simulink model "task2_3"  (R2015b)
settings: Solver=ode45  StartTime=tstart  StopTime=tstop  RelTol=1e-3
values from neighbouring files (symbols this model uses):
  c = 0    [matlab.mat]    (also in run.m; run_2_3.m = 1; test.m)
  delta_max = 0.436332312999    [matlab.mat]
  DELTA_s = 0.01    [matlab.mat]    (also in run_2_3.m = 1)
  k_b0 = 0.009    [matlab.mat]
  kd_psi = 500    [matlab.mat]
  ki_psi = 0.8    [matlab.mat]
  Ki_u = 0.0005    [matlab.mat]
  kp_psi = 190    [matlab.mat]
  Kp_u = 10    [matlab.mat]
  n_c_k = 1.02    [matlab.mat]
  n_c_max = 8.9    [matlab.mat]
  n_dot_max = 0.0436332312999    [matlab.mat]
  psi0 = 0    [matlab.mat]    (also in run.m; run_2_3.m; test.m)
  r0 = 0    [matlab.mat]    (also in run.m; run_2_3.m; test.m)
  tsamp = 10    [matlab.mat]    (also in run.m; run_2_3.m; test.m)
  Ua_MAX = 1    [matlab.mat]
  v0 = [6.63 0]    [matlab.mat]    (also in run.m = [6.63 0]'; run_2_3.m = [6.63 0]'; test.m = [6.63 0]')
  WP = [-600  4680  7662  10644  13626; 0  3880  2248  3878  2246]    [matlab.mat]
undefined symbols (not defined in the file or in its folder): Kd_u, msfartoystyring, N_u
undefined symbols (not defined in the file): p0
libraries: simulink x1
settings Model: ExtModeAutoUpdateStatusClock=off  Creator=christh  LastModifiedBy=ShivJeet
settings DataIOCC: SaveFormat=Array  SignalLoggingSaveFormat=ModelDataLogs
settings OptimizationCC: ExpressionDepthLimit=2147483647  InitFltsAndDblsToZero=on
settings DebuggingCC: UnderspecifiedInitializationDetection=Classic  MergeDetectMultiDrivingBlocksExec=none  SolverPrmCheckMsg=warning  FcnCallInpInsideContextMsg=UseLocalSettings  StateNameClashWarn=warning
settings HardwareCC: ProdBitPerPointer=32  ProdLargestAtomicFloat=None  ProdIntDivRoundTo=Undefined  ProdEndianess=Unspecified  ProdWordSize=32  ProdHWDeviceType=32-bit Generic
settings GRTTargetCC: GeneratePreprocessorConditionals=Disable all  CombineOutputUpdateFcns=off  GRTInterface=on
settings ConfigComp: CovModelRefEnable=Off

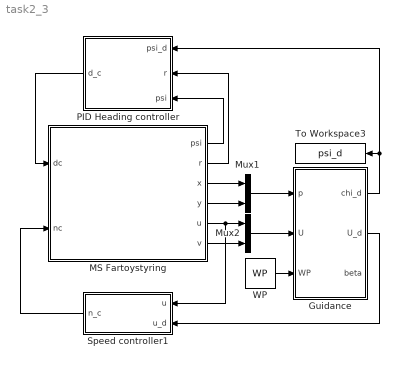
== system task2_3 ==
  Guidance : Subsystem
  MS Fartoystyring : Subsystem  mask(MS Fartoystyring for Assignment 3 G&C){x0=p0(1), y0=p0(2), u0=v0(1), v0=v0(2), psi0=psi0, r0=r0, c=c}
      mask prompts: x0 "x(t0) (m)"; y0 "y(t0) (m)"; u0 "u(t0) (m/s)"; v0 "v(t0) (m/s)"; psi0 "psi(t0) (rad)"; r0 "r(t0) (rad/s)"; c "current (0 or 1)"
      mask help:
      | Block corresponding to Figure 1 in the assignment text. Gives the response of the ship.
      |
      | The design speed of MS Fartoystyring is u=8.23 m/s.
      |
      | Input:
      | dc: commanded rudder (rad), dmax=25*pi/180
      | nc: commanded shaft speed (rad/s), nmax=85*2*pi/60
      |
      | Output:
      | x: north pos (m)
      | y: east pos (m)
      | u: surge (m/s)
      | v: sway (m/s)
      | psi: heading (rad)
      | r: yaw (rad/s)
      mask Help: Comments, bugs and help requests can be directed to the TA. Email on course website.
  Mux1 : Mux  Inputs=2
  Mux2 : Mux  Inputs=2
  PID Heading controller : Subsystem
  Speed controller1 : Subsystem
  To Workspace3 : ToWorkspace  VariableName=psi_d  SampleTime=tsamp
  WP : Constant  Value=WP
  wires:
  MS Fartoystyring/1(psi) -> PID Heading controller/3(psi)
  MS Fartoystyring/2(r) -> PID Heading controller/2(r)
  Speed controller1/1(n_c) -> MS Fartoystyring/2(nc)
  MS Fartoystyring/3(x) -> Mux1/1
  MS Fartoystyring/4(y) -> Mux1/2
  Mux1/1 -> Guidance/1(p)
  MS Fartoystyring/5(u) -> Speed controller1/1(u), Mux2/1
  PID Heading controller/1(d_c) -> MS Fartoystyring/1(dc)
  MS Fartoystyring/6(v) -> Mux2/2
  Mux2/1 -> Guidance/2(U)
  WP/1 -> Guidance/3(WP)
  Guidance/2(U_d) -> Speed controller1/2(u_d)
  Guidance/1(chi_d) -> PID Heading controller/1(psi_d), To Workspace3/1

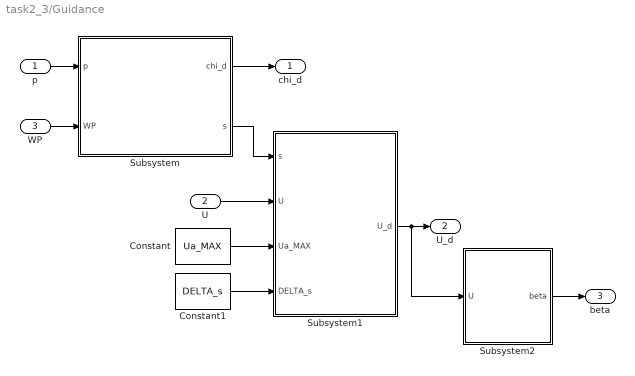
== system task2_3/Guidance ==
  p : Inport
  U : Inport  Port=2
  WP : Inport  Port=3
  Constant : Constant  Value=Ua_MAX
  Constant1 : Constant  Value=DELTA_s
  Subsystem : Subsystem
  Subsystem1 : Subsystem
  Subsystem2 : Subsystem
  chi_d : Outport
  U_d : Outport  Port=2
  beta : Outport  Port=3
  wires:
  U/1 -> Subsystem1/2("U ")
  Subsystem1/1(U_d) -> U_d/1, Subsystem2/1("U ")
  p/1 -> Subsystem/1(p)
  WP/1 -> Subsystem/2(WP)
  Subsystem/1(chi_d) -> chi_d/1
  Constant/1 -> Subsystem1/3(Ua_MAX)
  Subsystem/2(s) -> Subsystem1/1(s)
  Constant1/1 -> Subsystem1/4(DELTA_s)
  Subsystem2/1(beta) -> beta/1

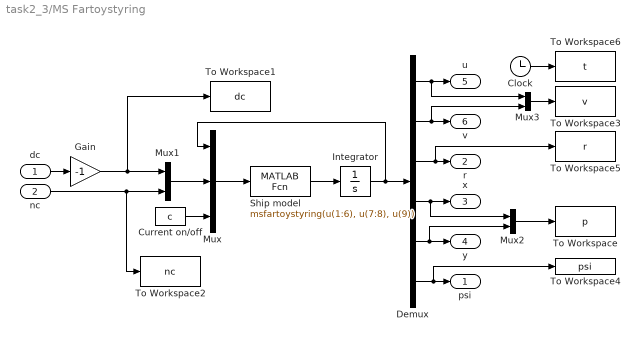
== system task2_3/MS Fartoystyring ==
  dc : Inport
  nc : Inport  Port=2
  Clock : Clock
  Current on/off : Constant  Value=c
  Demux : Demux  Outputs=6
  Gain : Gain  Gain=-1
  Integrator : Integrator  InitialCondition=[u0 v0 r0 x0 y0 psi0]'
  Mux : Mux  Inputs=3
  Mux1 : Mux  Inputs=2
  Mux2 : Mux  Inputs=2
  Mux3 : Mux  Inputs=2
  Ship model : MATLABFcn  MATLABFcn=msfartoystyring(u(1:6), u(7:8), u(9))  OutputDimensions=6
  To Workspace : ToWorkspace  VariableName=p  SampleTime=tsamp
  To Workspace1 : ToWorkspace  VariableName=dc  SampleTime=tsamp
  To Workspace2 : ToWorkspace  VariableName=nc  SampleTime=tsamp
  To Workspace3 : ToWorkspace  VariableName=v  SampleTime=tsamp
  To Workspace4 : ToWorkspace  VariableName=psi  SampleTime=tsamp
  To Workspace5 : ToWorkspace  VariableName=r  SampleTime=tsamp
  To Workspace6 : ToWorkspace  VariableName=t  SampleTime=tsamp
  psi : Outport
  r : Outport  Port=2
  x : Outport  Port=3
  y : Outport  Port=4
  u : Outport  Port=5
  v : Outport  Port=6
  wires:
  Integrator/1 -> Mux/1, Demux/1
  Mux1/1 -> Mux/2
  dc/1 -> Gain/1
  nc/1 -> Mux1/2, To Workspace2/1
  Demux/1 -> Mux3/1, u/1
  Demux/2 -> Mux3/2, v/1
  Demux/3 -> To Workspace5/1, r/1
  Demux/4 -> Mux2/1, x/1
  Demux/5 -> y/1, Mux2/2
  Demux/6 -> To Workspace4/1, psi/1
  Current on/off/1 -> Mux/3
  Ship model/1 -> Integrator/1
  Mux/1 -> Ship model/1
  Mux2/1 -> To Workspace/1
  Clock/1 -> To Workspace6/1
  Mux3/1 -> To Workspace3/1
  Gain/1 -> To Workspace1/1, Mux1/1

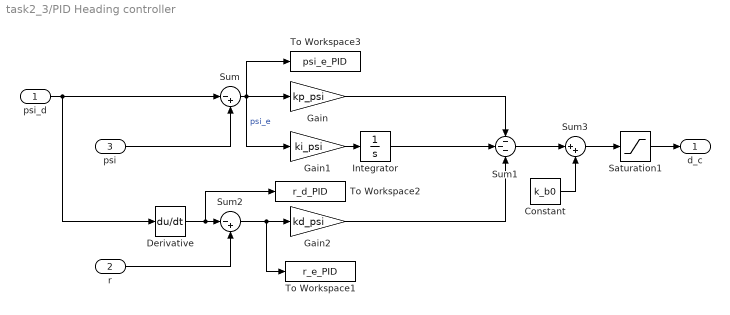
== system task2_3/PID Heading controller ==
  psi_d : Inport
  r : Inport  Port=2
  psi : Inport  Port=3
  Constant : Constant  Value=k_b0
  Derivative : Derivative
  Gain : Gain  Gain=kp_psi
  Gain1 : Gain  Gain=ki_psi
  Gain2 : Gain  Gain=kd_psi
  Integrator : Integrator
  Saturation1 : Saturate  UpperLimit=delta_max  LowerLimit=-delta_max
  Sum : Sum  Inputs=|-+
  Sum1 : Sum  Inputs=---
  Sum2 : Sum  Inputs=|-+
  Sum3 : Sum  Inputs=|++
  To Workspace1 : ToWorkspace  VariableName=r_e_PID  SampleTime=tsamp
  To Workspace2 : ToWorkspace  VariableName=r_d_PID  SampleTime=tsamp
  To Workspace3 : ToWorkspace  VariableName=psi_e_PID  SampleTime=tsamp
  d_c : Outport
  wires:
  psi_d/1 -> Derivative/1, Sum/1
  Saturation1/1 -> d_c/1
  Sum3/1 -> Saturation1/1
  psi/1 -> Sum/2
  Sum/1 -> Gain1/1, Gain/1, To Workspace3/1  "psi_e"
  Gain1/1 -> Integrator/1
  Gain/1 -> Sum1/1
  Integrator/1 -> Sum1/2
  Gain2/1 -> Sum1/3
  Sum1/1 -> Sum3/1
  Constant/1 -> Sum3/2
  Sum2/1 -> To Workspace1/1, Gain2/1
  r/1 -> Sum2/2
  Derivative/1 -> To Workspace2/1, Sum2/1

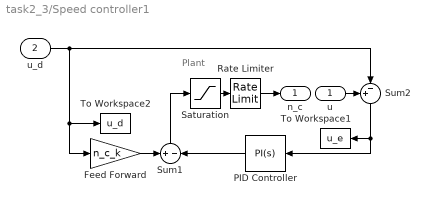
== system task2_3/Speed controller1 ==
  note: Plant
  u : Inport
  u_d : Inport  Port=2
  Feed Forward : Gain  Gain=n_c_k
  PID Controller : simulink/Continuous/PID Controller  Controller=PI  TimeDomain=Continuous-time  SampleTime=-1  IntegratorMethod=Forward Euler  FilterMethod=Forward Euler  Form=Parallel  UseFilter=on  ControllerParametersSource=internal  P=Kp_u  I=Ki_u  D=Kd_u  N=N_u  InitialConditionSource=internal  InitialConditionForIntegrator=0  InitialConditionForFilter=0  ExternalReset=none  LimitOutput=off  UpperSaturationLimit=inf  LowerSaturationLimit=-inf  LinearizeAsGain=on  AntiWindupMode=none  Kb=1  TrackingMode=off  Kt=1  PParamMin=[]  PParamMax=[]  IParamMin=[]  IParamMax=[]  DParamMin=[]  DParamMax=[]  NParamMin=[]  NParamMax=[]  KbParamMin=[]  KbParamMax=[]  KtParamMin=[]  KtParamMax=[]  POutMin=[]  POutMax=[]  IOutMin=[]  IOutMax=[]  DOutMin=[]  DOutMax=[]  NOutMin=[]  NOutMax=[]  KbOutMin=[]  KbOutMax=[]  KtOutMin=[]  KtOutMax=[]  IntegratorOutMin=[]  IntegratorOutMax=[]  FilterOutMin=[]  FilterOutMax=[]  SumOutMin=[]  SumOutMax=[]  SumI1OutMin=[]  SumI1OutMax=[]  SumI2OutMin=[]  SumI2OutMax=[]  SumI3OutMin=[]  SumI3OutMax=[]  SumDOutMin=[]  SumDOutMax=[]  SaturationOutMin=[]  SaturationOutMax=[]  IntegratorContinuousStateAttributes=''  IntegratorStateMustResolveToSignalObject=off  IntegratorRTWStateStorageClass=Auto  FilterContinuousStateAttributes=''  FilterStateMustResolveToSignalObject=off  FilterRTWStateStorageClass=Auto  DifferentiatorICPrevScaledInput=0  DifferentiatorOutMin=[]  DifferentiatorOutMax=[]
  Rate Limiter : RateLimiter  RisingSlewLimit=n_dot_max  FallingSlewLimit=-n_dot_max
  Saturation : Saturate  UpperLimit=n_c_max  LowerLimit=0.0001
  Sum1 : Sum  Inputs=+-
  Sum2 : Sum  Inputs=+-|
  To Workspace1 : ToWorkspace  VariableName=u_e  SampleTime=tsamp
  To Workspace2 : ToWorkspace  VariableName=u_d  SampleTime=tsamp
  n_c : Outport
  wires:
  Sum1/1 -> Saturation/1
  Saturation/1 -> Rate Limiter/1
  Rate Limiter/1 -> n_c/1
  u_d/1 -> Sum2/2, To Workspace2/1, Feed Forward/1
  Feed Forward/1 -> Sum1/1
  u/1 -> Sum2/1
  Sum2/1 -> PID Controller/1, To Workspace1/1
  PID Controller/1 -> Sum1/2

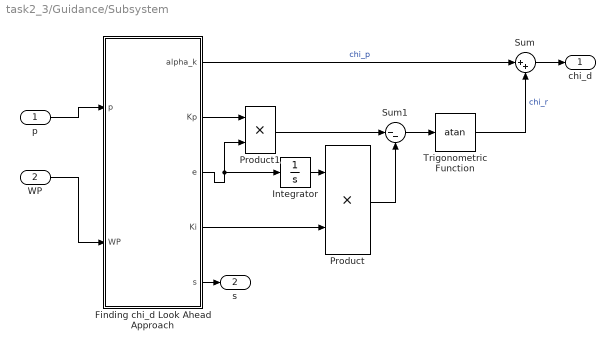
== system task2_3/Guidance/Subsystem ==
  p : Inport
  WP : Inport  Port=2
  Finding chi_d Look Ahead Approach : MATLAB Function  TreatAsAtomicUnit=on
  Integrator : Integrator
  Product : Product
  Product1 : Product
  Sum : Sum  Inputs=|++
  Sum1 : Sum  Inputs=|--
  Trigonometric Function : Trigonometry  Operator=atan
  chi_d : Outport
  s : Outport  Port=2
  wires:
  WP/1 -> Finding chi_d Look Ahead Approach/2(WP)
  p/1 -> Finding chi_d Look Ahead Approach/1(p)
  Sum1/1 -> Trigonometric Function/1
  Finding chi_d Look Ahead Approach/2(Kp) -> Product1/1
  Finding chi_d Look Ahead Approach/3(e) -> Product1/2, Integrator/1
  Integrator/1 -> Product/1
  Finding chi_d Look Ahead Approach/4(Ki) -> Product/2
  Finding chi_d Look Ahead Approach/1(alpha_k) -> Sum/1  "chi_p"
  Product1/1 -> Sum1/1
  Trigonometric Function/1 -> Sum/2  "chi_r"
  Product/1 -> Sum1/2
  Sum/1 -> chi_d/1
  Finding chi_d Look Ahead Approach/5(s) -> s/1

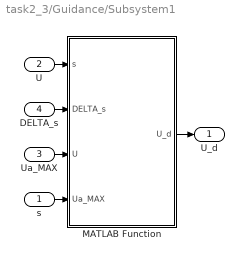
== system task2_3/Guidance/Subsystem1 ==
  s : Inport
  "U " : Inport  Port=2
  Ua_MAX : Inport  Port=3
  DELTA_s : Inport  Port=4
  MATLAB Function : MATLAB Function  TreatAsAtomicUnit=on
  U_d : Outport
  wires:
  "U "/1 -> MATLAB Function/1(s)
  DELTA_s/1 -> MATLAB Function/2(DELTA_s)
  Ua_MAX/1 -> MATLAB Function/3(U)
  s/1 -> MATLAB Function/4(Ua_MAX)
  MATLAB Function/1(U_d) -> U_d/1

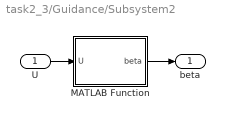
== system task2_3/Guidance/Subsystem2 ==
  "U " : Inport
  MATLAB Function : MATLAB Function  TreatAsAtomicUnit=on
  beta : Outport
  wires:
  "U "/1 -> MATLAB Function/1(U)
  MATLAB Function/1(beta) -> beta/1

== matlab function task2_3/Guidance/Subsystem1/MATLAB Function ==
  data: s input; DELTA_s input; U input; U_d output; Ua_MAX input
function U_d = fcn(s, DELTA_s, U, Ua_MAX)
%#codegen
U_t = sqrt(U(1)^2 + U(2)^2);

U_d = U_t - Ua_MAX * s/sqrt(s^2 + DELTA_s^2);
end

== matlab function task2_3/Guidance/Subsystem/Finding chi_d Look Ahead Approach ==
  data: p input; alpha_k output; WP input; Kp output; e output; Ki output; s output
function [alpha_k, Kp, e, Ki,s] = fcn(p, WP)

persistent index;

if isempty(index)
     index = 2;
end





%%
% The craft's position in NED
x = p(1);   %[m] 
y = p(2);   %[m]    



% The next and previous waypoint in NED
xk = WP(1, index - 1);                  xk_1 = WP(1, index); 
yk = WP(2, index - 1);                  yk_1 = WP(2, index);

% THE LOOKAHEAD DISTANCE R %%CHANGE THIS LATER
R = 1000;%sqrt((xk_1 - x)^2 + (yk_1 - y)^2);

% How far from the desired waypoint the craft must be before going to next
% waypoint
turning_Radius = 660; 

if (((xk_1 - x)^2 + (yk_1 - y)^2) <= turning_Radius^2) && (length(WP) > index)  
    index = index + 1;
end



%The angle between the North and two waypoints --> atan2(dy/dx)
alpha_k =  atan2(yk_1 - yk, xk_1 - xk); %[rad] 

%The rotation from the NED frame to path-fixed reference frame
Rp = [  cos(alpha_k)   -sin(alpha_k);
        sin(alpha_k)   cos(alpha_k);];
    
%How far the craft is from the previous way point
p_tilde = [x,y]' - [xk,yk]' % or p-WP_previous

% The coordinates of the craft in the path-fixed reference frame (Fossen
% p258)
Epsilon = Rp' * p_tilde;

% Along track distance & cross track error
s = Epsilon(1,:);
e = Epsilon(2,:);

%The look ahead distance DELTA
DELTA = sqrt(R^2-e^2);
disp('-e/DELTA')
disp(atan(-e/DELTA))
disp('alpha')
disp(alpha_k)
% Steering law
Kp = 1/DELTA;
Ki = 0;
end

== matlab function task2_3/Guidance/Subsystem2/MATLAB Function ==
  data: U input; beta output
function beta = fcn(U)
%#codegen
u = U(1);
v = U(2);

beta = asin(v/sqrt(u^2 +v^2));
end;
